simulink model "ME419TermProj"  (R2023b)
settings: Solver=VariableStepAuto  StartTime=0.0  StopTime=50  RelTol=1e-9
undefined symbols (not defined in the file): b, J, K_d, K_i, K_p, K_v, Ka, L, R
settings Model: Creator=Aiden  LastModifiedBy=julia

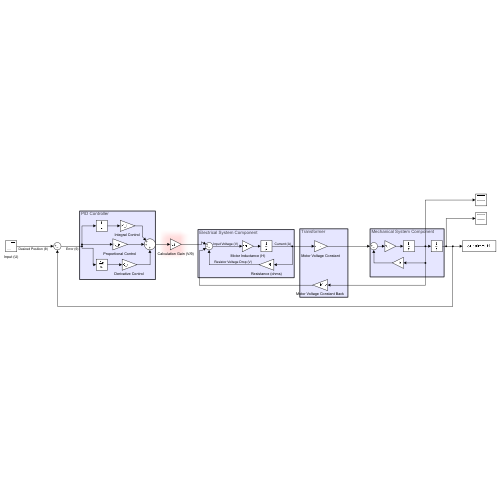
[thumbnail: Simulink's stored preview of the top-level diagram]
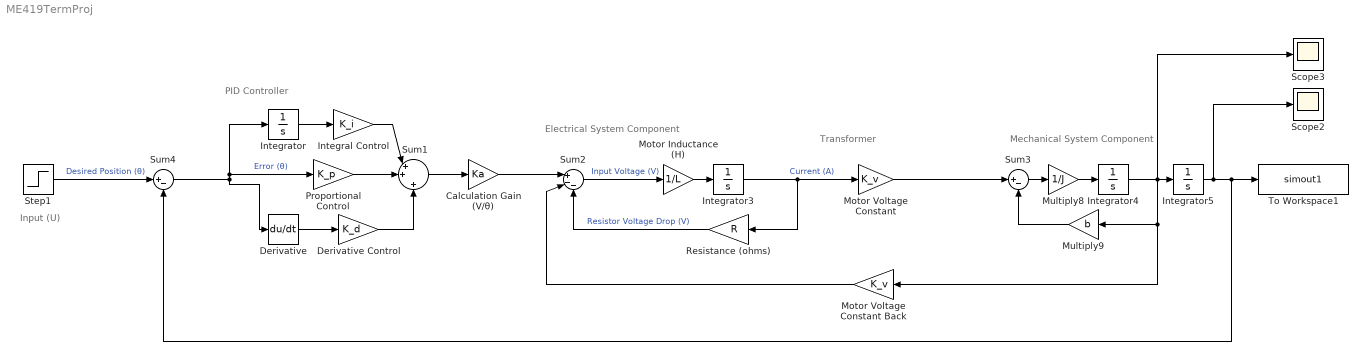
== system ME419TermProj ==
  note: Input (U)
  note: Electrical System Component
  note: PID Controller
  note: Transformer
  note: Mechanical System Component
  Calculation Gain (V/θ) : Gain  Gain=Ka
  Derivative : Derivative
  "Derivative Control " : Gain  Gain=K_d
  "Integral Control " : Gain  Gain=K_i
  Integrator{,3..5} (4 alike) : Integrator
  Motor Inductance (H) : Gain  Gain=1/L
  "Motor Voltage Constant " : Gain  Gain=K_v
  Motor Voltage Constant Back : Gain  Gain=K_v
  Multiply8 : Gain  Gain=1/J
  Multiply9 : Gain  Gain=b
  "Proportional Control " : Gain  Gain=K_p
  Resistance (ohms) : Gain  Gain=R
  Scope2 : Scope
  Scope3 : Scope
  Step1 : Step  SampleTime=0
  Sum1 : Sum  Inputs=|++|+
  Sum2 : Sum  Inputs=|+--
  Sum3 : Sum  Inputs=|+-
  Sum4 : Sum  Inputs=|+-
  To Workspace1 : ToWorkspace  VariableName=simout1  SampleTime=-1
  wires:
  Motor Voltage Constant Back/1 -> Sum2/2
  Resistance (ohms)/1 -> Sum2/3  "Resistor Voltage Drop (V)"
  Multiply9/1 -> Sum3/2
  Multiply8/1 -> Integrator4/1
  Sum3/1 -> Multiply8/1
  "Motor Voltage Constant "/1 -> Sum3/1
  Integrator3/1 -> Resistance (ohms)/1, "Motor Voltage Constant "/1  "Current (A)"
  Integrator4/1 -> Scope3/1, Multiply9/1, Motor Voltage Constant Back/1, Integrator5/1
  Sum2/1 -> Motor Inductance (H)/1  "Input Voltage (V)"
  Motor Inductance (H)/1 -> Integrator3/1
  Step1/1 -> Sum4/1  "Desired Position (θ)"
  Integrator5/1 -> Sum4/2, To Workspace1/1, Scope2/1
  Sum4/1 -> Derivative/1, Integrator/1, "Proportional Control "/1  "Error (θ)"
  Integrator/1 -> "Integral Control "/1
  Derivative/1 -> "Derivative Control "/1
  Sum1/1 -> Calculation Gain (V/θ)/1
  "Proportional Control "/1 -> Sum1/2
  "Integral Control "/1 -> Sum1/1
  "Derivative Control "/1 -> Sum1/3
  Calculation Gain (V/θ)/1 -> Sum2/1
